simulink model "vardownsampler"  (Simulink 7.3)
settings: Solver=VariableStepDiscrete  StartTime=0.0  StopTime=simTime*SampleTime  RelTol=1e-3
PreLoadFcn:
  | setup_vardownsampler
InitFcn:
  | setup_vardownsampler
values from neighbouring files (symbols this model uses):
  accumOutShift = [1 4 3 2 4]    [setup_vardownsampler.m]    (also in setup_vardownsamplerL8.m = [3 3 2 2 2])
  accumOutWidth = dataWidth + ceil(log2(Rmax))+0    [setup_vardownsampler.m]    (also in setup_vardownsamplerL8.m)
  adderOutShift = 4*ones(1,numRates)    [setup_vardownsampler.m]    (also in setup_vardownsamplerL8.m = 3*ones(1,numRates))
  adderOutWidth = dataWidth + coeffWidth + ceil(log2(L))    [setup_vardownsampler.m]    (also in setup_vardownsamplerL8.m)
  addrWidth = max(1,ceil(log2(Rmax)))    [setup_vardownsampler.m]    (also in setup_vardownsamplerL8.m)
  ChanCount = 16    [setup_vardownsampler.m]    (also in setup_vardownsamplerL8.m = 1)
  ChanCycleCount = ceil(ChanCount/ChanWireCount)    [setup_vardownsampler.m]    (also in setup_vardownsamplerL8.m)
  ChanWireCount = ceil(ChanCount/Period)    [setup_vardownsampler.m]    (also in setup_vardownsamplerL8.m)
  coeffWidth = 16    [setup_vardownsampler.m]    (also in setup_vardownsamplerL8.m)
  dataWidth = 16    [setup_vardownsampler.m]    (also in setup_vardownsamplerL8.m)
  FirAddr = AccumOutScale + 1    (= 4)    [setup_vardownsampler.m]    (also in setup_vardownsamplerL8.m)
  hmatrix = zeros(2*Rmax, L)    [setup_vardownsampler.m]    (also in setup_vardownsamplerL8.m)
  memAddrWidth = max(1,ceil(log2(Nmax)))    [setup_vardownsampler.m]    (also in setup_vardownsamplerL8.m)
  Nmax = Period*Rmax    [setup_vardownsampler.m]    (also in setup_vardownsamplerL8.m)
  Period = floor(ClockRate / SampleRate)    [setup_vardownsampler.m]    (also in setup_vardownsamplerL8.m)
  R = [1 2 5 8 2]    [setup_vardownsampler.m]    (also in setup_vardownsamplerL8.m = [4 5 7 8 9])
  RateWidth = ceil(log2(Rmax))+1    [setup_vardownsampler.m]    (also in setup_vardownsamplerL8.m)
  resetCntWidth = max(1,ceil(log2(Nmax)))    [setup_vardownsampler.m]    (also in setup_vardownsamplerL8.m)
  Rmax = 16    [setup_vardownsampler.m]    (also in setup_vardownsamplerL8.m = 20)
  SampleTime = 1    [setup_vardownsampler.m]    (also in setup_vardownsamplerL8.m)
undefined symbols (not defined in the file or in its folder): AdvDSPBChannelOutDisplay, AdvDSPBDMemDisplay, bank1, bank2, c4, c5, c6, c7, c8, c9, dpoly, dspba_ChannelInVis, dspba_ChannelOutVis, dspba_internal_get_channel_ports, evalAionMaskParam, hmatrix0, hmatrix1, hmatrix2, hmatrix3, latency, primtype, UseDontCare, value
libraries: DSPBAPrim x314, DSPBAModelBus x24, simulink x12, DSPBABase x6
(part 1 of 4)
Description:
  | This model shows how to use the primitive blocks to build a variable integer rate decimation FIR filter. The model has the following features:
  | •Support arbitrary integer decimation rate (including the cases without rate change), arbitrary number of channels and arbitrary clock rate and input sample rate, as long as the clock rate is high enough to process all channels in a single data path (i.e. no hardware duplication).
  | •Support run time reconfiguration of decimation rate.
  | •Use of two memory banks for filter coefficients storage instead of pre-storing coefficients for all rates in memory.  Update one memory bank while the design is reading coefficients from the other bank.
  | •Real time control of scaling in the FIR data path.
  | 
  | The model will generate RTL that can be used in the third party tools.
  | 
  | The parameters for the system can be modified in the file setup_vardownsampleri.m which can be accessed from the Edit Params icon.
settings Model: Creator=sichou  LastModifiedBy=xdong
settings OptimizationCC: InitFltsAndDblsToZero=on
settings DebuggingCC: SaveWithParameterizedLinksMsg=none  SignalResolutionControl=TryResolveAllWithWarning  MultiTaskDSMMsg=warning  MultiTaskCondExecSysMsg=none  StrictBusMsg=None  LoggingUnavailableSignals=none
settings RTWCC: IncludeERTFirstTime=on
settings GRTTargetCC: TargetFcnLib=ansi_tfl_tmw.mat

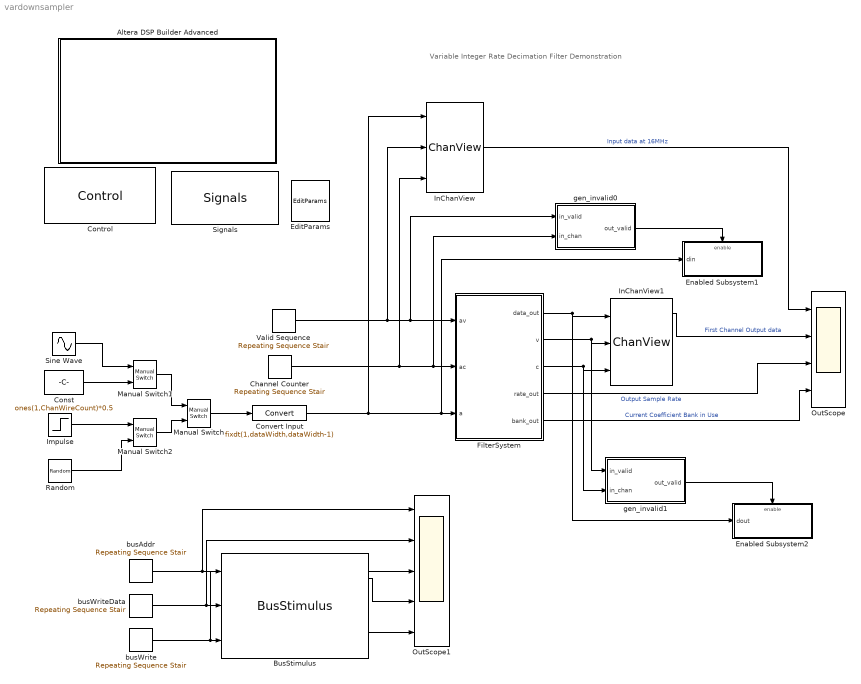
== system vardownsampler ==
  note: Variable Integer Rate Decimation Filter Demonstration
  Altera DSP Builder Advanced : Subsystem
      settings: OpenFcn=web('http://www.altera.com', '-new');
      mask Type: DSP Builder Advanced Blockset Ignored Block
      mask Display: image(imread('alteralogo.tif'));
  BusStimulus : DSPBAModelBus/BusStimulus  SampleTime=-1  version=20090407
  Channel Counter : simulink/Sources/Repeating Sequence Stair  SystemSampleTime=-1  OutValues=[0:ChanCycleCount-1 zeros(1,Period-ChanCycleCount)]  tsamp=SampleTime  OutMin=[]  OutMax=[]  OutDataTypeStr=uint(8)  OutputDataTypeScalingMode=Specify via dialog  OutDataType=uint(8)  ConRadixGroup=Best Precision: Vector-wise  OutScaling=2^-12
  Const : Constant  Value=ones(1,ChanWireCount)*0.5  OutDataType=sfix(16)  OutScaling=2^0
  Control : DSPBABase/Control  generate=off  destination=../rtl  language=VHDL  autotestbench=off  signaldepth=2  coveragetestbench=off  logs=off  spacewidth=2  spacenum=2  addrwidth=16  datawidth=32  dataendian=Big Endian  hierarchicalnames=on  ramThresholdBits=-1  distRamThresholdBits=-1  mlabThresholdBits=-1  hardMultiplierThresholdLuts=-1  version=20090407
  Convert Input : DataTypeConversion  OutDataTypeMode=Specify via dialog  OutDataType=fixdt(1,dataWidth,dataWidth-1)  OutDataTypeStr=fixdt(1,dataWidth,dataWidth-1)  SaturateOnIntegerOverflow=on
  EditParams : DSPBABase/EditParams  SystemSampleTime=-1  version=20090407
  Enabled Subsystem1 : Subsystem  TreatAsAtomicUnit=on
  Enabled Subsystem2 : Subsystem  TreatAsAtomicUnit=on
  FilterSystem : Subsystem
  Impulse : Step  Time=ones(1, ChanWireCount)  Before=1  After=0  SampleTime=SampleTime
  InChanView : DSPBABase/ChanView  nchans=ChanCount  chan_vector=0  latency=0  version=20090407
  InChanView1 : DSPBABase/ChanView  nchans=ChanCount  chan_vector=0:ChanCount-1  latency=0  version=20090407
  Manual Switch : simulink/Signal Routing/Manual Switch  SystemSampleTime=-1  sw=1  action=0  varsize=off
  Manual Switch1 : simulink/Signal Routing/Manual Switch  SystemSampleTime=-1  sw=1  action=0  varsize=off
  Manual Switch2 : simulink/Signal Routing/Manual Switch  SystemSampleTime=-1  sw=0  action=0  varsize=off
  OutScope : Scope  NumInputPorts=4
      settings: TimeRange=20000  YMin=-1~-0.5~-5~-5  YMax=1~0.5~5~5  SaveName=iout  DataFormat=Structure
  OutScope1 : Scope  NumInputPorts=5
      settings: TimeRange=20000  YMin=-1~-0.5~-5~-5~-5  YMax=1~0.5~5~5~5  SaveName=iout1  DataFormat=Structure
  Random : RandomNumber  Seed=1:ChanWireCount  SampleTime=SampleTime
  Signals : DSPBABase/Signals  SystemSampleTime=-1  clk=clk  freq=ClockRate  margin=ClockMargin  rst=areset  rstactive=High  bus=bus  enbusclock=on  busfreq=BusClockRate  bussync=on  version=20090407
  Sine Wave : Sin  SineType=Sample based  Amplitude=ones(1,ChanWireCount)*(2^17-2)/(2^17)  Bias=0  Frequency=(2 * pi) / ( 4 * 2^24 / floor(2^24 * 0.051))  Phase=0  Samples=Rmax*50  SampleTime=SampleTime  Offset=0
  Valid Sequence : simulink/Sources/Repeating Sequence Stair  SystemSampleTime=-1  OutValues=v_in  tsamp=SampleTime  OutMin=[]  OutMax=[]  OutDataTypeStr=Inherit: Inherit via back propagation  OutDataType=float('double')  ConRadixGroup=Best Precision: Vector-wise  OutScaling=2^-12
  busAddr : simulink/Sources/Repeating Sequence Stair  SystemSampleTime=-1  OutValues=busAddr  tsamp=SampleTime  OutMin=[]  OutMax=[]  OutDataTypeStr=uint16  OutputDataTypeScalingMode=uint16  OutDataType=float('double')  ConRadixGroup=Best Precision: Vector-wise  OutScaling=2^-12
  busWrite : simulink/Sources/Repeating Sequence Stair  SystemSampleTime=-1  OutValues=busWrite  tsamp=SampleTime  OutMin=[]  OutMax=[]  OutDataTypeStr=Inherit: Inherit via back propagation  OutDataType=ufix(1)  ConRadixGroup=Best Precision: Vector-wise  OutScaling=[]
  busWriteData : simulink/Sources/Repeating Sequence Stair  SystemSampleTime=-1  OutValues=busWriteData  tsamp=SampleTime  OutMin=[]  OutMax=[]  OutDataTypeStr=uint32  OutputDataTypeScalingMode=uint32  OutDataType=fixdt(1,32,2^0,0)  ConRadixGroup=Best Precision: Vector-wise  OutScaling=[]
  gen_invalid0 : Subsystem
  gen_invalid1 : Subsystem
  wires:
  Manual Switch2/1 -> Manual Switch/2
  Impulse/1 -> Manual Switch2/1
  Random/1 -> Manual Switch2/2
  Manual Switch/1 -> Convert Input/1
  Manual Switch1/1 -> Manual Switch/1
  Sine Wave/1 -> Manual Switch1/1
  Const/1 -> Manual Switch1/2
  Convert Input/1 -> InChanView/1, Enabled Subsystem1/1(din), FilterSystem/3(a)
  Channel Counter/1 -> InChanView/3, FilterSystem/2(ac), gen_invalid0/2(in_chan)
  Valid Sequence/1 -> InChanView/2, FilterSystem/1(av), gen_invalid0/1(in_valid)
  gen_invalid1/1(out_valid) -> Enabled Subsystem2/Enable
  gen_invalid0/1(out_valid) -> Enabled Subsystem1/Enable
  busAddr/1 -> BusStimulus/1, OutScope1/1
  busWriteData/1 -> BusStimulus/2, OutScope1/2
  busWrite/1 -> BusStimulus/3, OutScope1/3
  InChanView/1 -> OutScope/1  "Input data at 16MHz"
  InChanView1/1 -> OutScope/2  "First Channel Output data"
  BusStimulus/1 -> OutScope1/4
  BusStimulus/2 -> OutScope1/5
  FilterSystem/1(data_out) -> InChanView1/1, Enabled Subsystem2/1(dout)
  FilterSystem/2(v) -> InChanView1/2, gen_invalid1/1(in_valid)
  FilterSystem/3(c) -> InChanView1/3, gen_invalid1/2(in_chan)
  FilterSystem/4(rate_out) -> OutScope/3  "Output Sample Rate"
  FilterSystem/5(bank_out) -> OutScope/4  "Current Coefficient Bank in Use"

== system vardownsampler/Altera DSP Builder Advanced ==

== system vardownsampler/Enabled Subsystem1 ==
  din : Inport  OutDataType=fixdt(1, 16)  OutScaling=2^0
  Enable : EnablePort
  To Workspace : ToWorkspace  VariableName=din  SampleTime=SampleTime  SaveFormat=Array
  wires:
  din/1 -> To Workspace/1

== system vardownsampler/Enabled Subsystem2 ==
  dout : Inport  OutDataType=fixdt(1, 16)  OutScaling=2^0
  Enable : EnablePort
  To Workspace : ToWorkspace  VariableName=dout  SampleTime=SampleTime  SaveFormat=Array
  wires:
  dout/1 -> To Workspace/1

== system vardownsampler/FilterSystem ==
  av : Inport  OutDataType=sfix(16)  OutScaling=2^0
  ac : Inport  Port=2  OutDataType=sfix(16)  OutScaling=2^0
  a : Inport  Port=3  OutDataType=sfix(16)  OutScaling=2^0
  Device : DSPBABase/Device  SystemSampleTime=-1  family=Stratix IV  deviceMember=Stratix IV E  stratix4device=Stratix IV E  hardcopy4device=HardCopy IV E  device=AUTO  speed=-2  stratixSpeed=-5  stratix2Speed=-3  stratix3Speed=-2  stratix4gxSpeed=-2  stratix4gtSpeed=-1  cyclone2Speed=-6  cyclone3Speed=-6  arria2Speed=-4  ecp2Speed=-7  version=20090914
  FIRSubsystem : Subsystem
  Rate : DSPBAModelBus/RegField  reg_name=RateAddr  reg_rwmode=Read/Write  reg_msb=RateWidth-1  reg_lsb=0  reg_type=ufix(RateWidth)  reg_scale=1  reg_init=R(1)  reg_desc=Decimation Rate  reg_modal=off  reg_desc0=0  reg_desc1=0  reg_desc2=0  reg_desc3=0  reg_desc4=0  reg_desc5=0  reg_desc6=0  reg_desc7=0  reg_addr=1  SampleTime=SampleTime  version=20090407
  Terminator : Terminator
  coefficients_gen : Subsystem
  gen_addr_control : Subsystem
  data_out : Outport  OutDataType=sfix(16)  OutScaling=2^0
  v : Outport  Port=2  OutDataType=sfix(16)  OutScaling=2^0
  c : Outport  Port=3  OutDataType=sfix(16)  OutScaling=2^0
  rate_out : Outport  Port=4  OutDataType=sfix(16)  OutScaling=2^0
  bank_out : Outport  Port=5  OutDataType=sfix(16)  OutScaling=2^0
  wires:
  Rate/1 -> gen_addr_control/3(rate_in)
  av/1 -> gen_addr_control/1(v)
  ac/1 -> gen_addr_control/2(c)
  a/1 -> gen_addr_control/4(data_in)
  gen_addr_control/1(qv) -> coefficients_gen/1(v)
  gen_addr_control/2(qc) -> coefficients_gen/2(c)
  gen_addr_control/3(coeff_addr) -> coefficients_gen/3(coeff_addr)
  coefficients_gen/3(coeff) -> FIRSubsystem/3(coeff)
  coefficients_gen/1(qv) -> FIRSubsystem/1(dv)
  coefficients_gen/2(qc) -> FIRSubsystem/2(dc)
  gen_addr_control/5(mem_addr) -> coefficients_gen/5(mem_addr)
  gen_addr_control/6(data_out) -> coefficients_gen/6(data_in)
  gen_addr_control/7(rate_out) -> coefficients_gen/7(rate_in)
  gen_addr_control/8(outvalid) -> coefficients_gen/8(outvalid_in)
  coefficients_gen/4(mem_addr_out) -> FIRSubsystem/4(mem_addr)
  coefficients_gen/5(data_out) -> FIRSubsystem/5(data_in)
  coefficients_gen/6(rate_out) -> FIRSubsystem/6(rate_in)
  coefficients_gen/7(outvalid) -> FIRSubsystem/7(outvalid_in)
  FIRSubsystem/4(rate_out) -> rate_out/1
  FIRSubsystem/3(data_out) -> data_out/1
  FIRSubsystem/2(c) -> c/1
  FIRSubsystem/5(valid_out) -> v/1
  FIRSubsystem/1(v) -> Terminator/1
  gen_addr_control/4(coffset) -> coefficients_gen/4(coffset)
  coefficients_gen/8(bank) -> FIRSubsystem/8(bank_in)
  FIRSubsystem/6(bank_out) -> bank_out/1

== system vardownsampler/gen_invalid0 ==
  note: Generate valid signal for the 1st channel
  in_valid : Inport
  in_chan : Inport  Port=2
  Bitwise Operator : simulink/Logic and Bit Operations/Bitwise Operator  logicop=AND  UseBitMask=off  NumInputPorts=2  BitMask=bin2dec('11011001')  BitMaskRealWorld=Stored Integer
  Compare To Constant : simulink/Logic and Bit Operations/Compare To Constant  SystemSampleTime=-1  relop===  const=0  LogicOutDataTypeMode=boolean  ZeroCross=off
  out_valid : Outport
  wires:
  Compare To Constant/1 -> Bitwise Operator/2
  in_valid/1 -> Bitwise Operator/1
  in_chan/1 -> Compare To Constant/1
  Bitwise Operator/1 -> out_valid/1

== system vardownsampler/gen_invalid1 ==
  note: Generate valid signal for the 1st channel
  in_valid : Inport
  in_chan : Inport  Port=2
  Bitwise Operator : simulink/Logic and Bit Operations/Bitwise Operator  logicop=AND  UseBitMask=off  NumInputPorts=2  BitMask=bin2dec('11011001')  BitMaskRealWorld=Stored Integer
  Compare To Constant : simulink/Logic and Bit Operations/Compare To Constant  SystemSampleTime=-1  relop===  const=0  LogicOutDataTypeMode=boolean  ZeroCross=off
  out_valid : Outport
  wires:
  in_chan/1 -> Compare To Constant/1
  Compare To Constant/1 -> Bitwise Operator/2
  in_valid/1 -> Bitwise Operator/1
  Bitwise Operator/1 -> out_valid/1

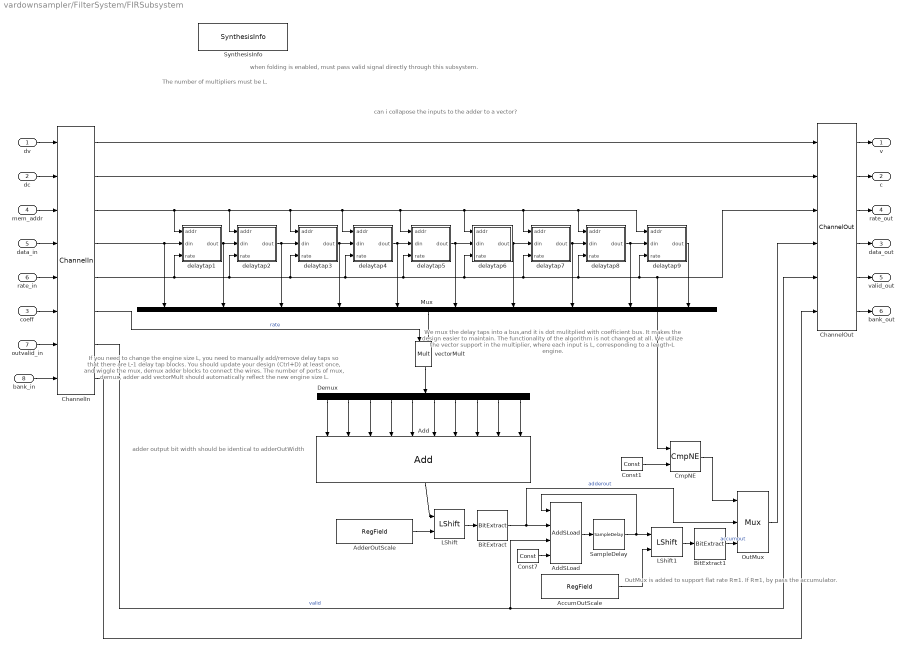
== system vardownsampler/FilterSystem/FIRSubsystem ==
  note: adder output bit width should be identical to adderOutWidth
  note: when folding is enabled, must pass valid signal directly through this subsystem.
  note: The number of multipliers must be L.
  note: can i collapose the inputs to the adder to a vector?
  note: We mux the delay taps into a bus,and it is dot mulitplied
      | with coefficient bus.  It makes the design easier to maintain.
      | The functionality of the algorithm is not changed at all.
      | We utilize the vector support in the multiplier, where
      | each input is L, corresponding to a length-L engine.
  note: If you need to change the engine size L,
      | you need to manually add/remove delay taps
      | so that there are L-1 delay tap blocks.  You should
      | update your design (Ctrl+D) at least once, and
      | wiggle the mux, demux adder blocks to connect
      |  the wires.  The number of ports of mux, demux, adder
      | add vectorMult should automatically reflect the new
      | engine size L.
  note: OutMux is added to support flat rate R=1.
      | If R=1, by pass the accumulator.
  dv : Inport  OutDataType=sfix(16)  OutScaling=2^0
  dc : Inport  Port=2  OutDataType=sfix(16)  OutScaling=2^0
  coeff : Inport  Port=3  OutDataType=sfix(16)  OutScaling=2^0
  mem_addr : Inport  Port=4  OutDataType=sfix(16)  OutScaling=2^0
  data_in : Inport  Port=5  OutDataType=sfix(16)  OutScaling=2^0
  rate_in : Inport  Port=6  OutDataType=sfix(16)  OutScaling=2^0
  outvalid_in : Inport  Port=7  OutDataType=sfix(16)  OutScaling=2^0
  bank_in : Inport  Port=8  OutDataType=sfix(16)  OutScaling=2^0
  AccumOutScale : DSPBAModelBus/RegField  reg_name=AccumOutScale  reg_rwmode=Read/Write  reg_msb=15  reg_lsb=0  reg_type=ufix(16)  reg_scale=1  reg_init=accumOutShift(1)  reg_desc=Left shift value forthe final accumulator output  reg_modal=off  reg_desc0=0  reg_desc1=0  reg_desc2=0  reg_desc3=0  reg_desc4=0  reg_desc5=0  reg_desc6=0  reg_desc7=0  reg_addr=3  SampleTime=-1  version=20090407
  Add : DSPBAPrim/Add  primtype=add  nInputs=evalAionMaskParam(gcb,'value',1)  nOutputs=1  omode=Inherit via internal rule with word growth  otype=sfix(adderOutWidth)  scale=2^-(adderOutWidth-1)  rndmethod=Unbiased  factor=1  satmethod=Symmetric  shift_vec=[0 1 2 -1]  value=L  inPortNames=[' '; ' ';]  outPortNames=[' ']  image=dspba_prim.jpg  text=fprintf('+');  style=Optimised  visibilities=1032  version=20090731
  AddSLoad : DSPBAPrim/AddSLoad  primtype=addsload  nInputs=4  nOutputs=1  omode=Specify via dialog  otype=sfix(accumOutWidth)  scale=2^-(dataWidth-1)  rndmethod=Unbiased  factor=1  satmethod=Symmetric  shift_vec=[0 1 2 -1]  value=0  inPortNames=['+'; '+'; 's'; 'v']  outPortNames=[' ']  image=dspba_prim.jpg  text=fprintf('+');  style=Optimised  visibilities=8  version=20090407
  AdderOutScale : DSPBAModelBus/RegField  reg_name=AdderOutScale  reg_rwmode=Read/Write  reg_msb=15  reg_lsb=0  reg_type=ufix(16)  reg_scale=1  reg_init=adderOutShift(1)  reg_desc=Left shift value forthe final adder output  reg_modal=off  reg_desc0=0  reg_desc1=0  reg_desc2=0  reg_desc3=0  reg_desc4=0  reg_desc5=0  reg_desc6=0  reg_desc7=0  reg_addr=2  SampleTime=-1  version=20090407
  BitExtract : DSPBAPrim/BitExtract  primtype=bitextract  nInputs=1  nOutputs=1  omode=Specify via dialog  otype=sfix(dataWidth)  scale=2^-(dataWidth-1)  rndmethod=Unbiased  factor=1  satmethod=Symmetric  shift_vec=[0 1 2 -1]  value=adderOutWidth - dataWidth  inPortNames=[' '; ' ';]  outPortNames=[' ']  image=dspba_prim.jpg  text=fprintf('..%d', value);  style=Optimised  visibilities=8 + 1024  version=20090407
  BitExtract1 : DSPBAPrim/BitExtract  primtype=bitextract  nInputs=1  nOutputs=1  omode=Specify via dialog  otype=sfix(dataWidth)  scale=2^-(dataWidth-1)  rndmethod=Unbiased  factor=1  satmethod=Symmetric  shift_vec=[0 1 2 -1]  value=accumOutWidth - dataWidth  inPortNames=[' '; ' ';]  outPortNames=[' ']  image=dspba_prim.jpg  text=fprintf('..%d', value);  style=Optimised  visibilities=8 + 1024  version=20090407
  ChannelIn : DSPBAPrim/ChannelIn  primtype=channelin  nInputs=dspba_internal_get_channel_ports(gcb)  nOutputs=dspba_internal_get_channel_ports(gcb)  omode=Inherit via internal rule  otype=sfix(16)  scale=2^-15  rndmethod=Unbiased  factor=1  satmethod=Symmetric  shift_vec=[0 1 2 -1]  value=6  inPortNames=['v'; 'c'; '0'; '1'; '2'; '3'; '4'; '5'; '6'; '7'; '8'; '9'; 'A'; 'B'; 'D'; 'E'; 'F'; 'G'; 'H'; 'I'; 'J'; 'K'; 'L'; 'M'; 'N'; 'O'; 'P'; 'Q'; 'R'; 'S'; 'T'; 'U'; 'W'; 'X'; 'Y'; 'Z']  outPortNames=['v'; 'c'; '0'; '1'; '2'; '3'; '4'; '5'; '6'; '7'; '8'; '9'; 'A'; 'B'; 'D'; 'E'; 'F'; 'G'; 'H'; 'I'; 'J'; 'K'; 'L'; 'M'; 'N'; 'O'; 'P'; 'Q'; 'R'; 'S'; 'T'; 'U'; 'W'; 'X'; 'Y'; 'Z']  image=dspba_prim.jpg  text=fprintf('In');  style=Optimised  dataSignals=6  foldingEnabled=off  channels=ChanCount  sampleRate=SampleRate  visibilities=dspba_ChannelInVis(gcb)  version=20090408
  ChannelOut : DSPBAPrim/ChannelOut  primtype=channelout  nInputs=dspba_internal_get_channel_ports(gcb)  nOutputs=dspba_internal_get_channel_ports(gcb)  omode=Inherit via internal rule  otype=sfix(16)  scale=2^-15  rndmethod=Unbiased  factor=1  satmethod=Symmetric  shift_vec=[0 1 2 -1]  value=4  inPortNames=['v'; 'c'; '0'; '1'; '2'; '3'; '4'; '5'; '6'; '7'; '8'; '9'; 'A'; 'B'; 'D'; 'E'; 'F'; 'G'; 'H'; 'I'; 'J'; 'K'; 'L'; 'M'; 'N'; 'O'; 'P'; 'Q'; 'R'; 'S'; 'T'; 'U'; 'W'; 'X'; 'Y'; 'Z']  outPortNames=['v'; 'c'; '0'; '1'; '2'; '3'; '4'; '5'; '6'; '7'; '8'; '9'; 'A'; 'B'; 'D'; 'E'; 'F'; 'G'; 'H'; 'I'; 'J'; 'K'; 'L'; 'M'; 'N'; 'O'; 'P'; 'Q'; 'R'; 'S'; 'T'; 'U'; 'W'; 'X'; 'Y'; 'Z']  image=dspba_prim.jpg  text=fprintf('Out%s', AdvDSPBChannelOutDisplay(latency));  style=Optimised  dataSignals=4  foldingEnabled=off  channels=ChanCount  sampleRate=SampleRate  visibilities=dspba_ChannelOutVis(gcb)  latency=0  version=20090408
  CmpNE : DSPBAPrim/CmpNE  primtype=cmpne  nInputs=2  nOutputs=1  omode=boolean  otype=sfix(16)  scale=2^-15  rndmethod=Unbiased  factor=1  satmethod=Symmetric  shift_vec=[0 1 2 -1]  value=0  inPortNames=[' '; ' ';]  outPortNames=[' ']  image=dspba_prim.jpg  text=fprintf('~=');  style=Optimised  visibilities=0  version=20090407
  Const1 : DSPBAPrim/Const  primtype=const  nInputs=0  nOutputs=1  omode=Specify via dialog  otype=ufix(RateWidth)  scale=1  rndmethod=Unbiased  factor=1  satmethod=Symmetric  shift_vec=[0 1 2 -1]  value=1  inPortNames=['+'; '+';]  outPortNames=[' ']  image=dspba_prim.jpg  text=fprintf('%s', num2str(value));  style=Optimised  visibilities=8 + 1024  version=20090407
  Const7 : DSPBAPrim/Const  primtype=const  nInputs=0  nOutputs=1  omode=Specify via dialog  otype=uint(accumOutWidth)  scale=1  rndmethod=Unbiased  factor=1  satmethod=Symmetric  shift_vec=[0 1 2 -1]  value=0  inPortNames=['+'; '+';]  outPortNames=[' ']  image=dspba_prim.jpg  text=fprintf('%s', num2str(value));  style=Optimised  visibilities=8 + 1024  version=20090407
  Demux : Demux  Outputs=L
  LShift : DSPBAPrim/LShift  primtype=lshift  nInputs=2  nOutputs=1  omode=Specify via dialog  otype=sfix(adderOutWidth)  scale=1  rndmethod=Unbiased  factor=1  satmethod=Symmetric  shift_vec=[0 1 2 -1]  value=0  inPortNames=['a'; 'b';]  outPortNames=[' ']  image=dspba_prim.jpg  text=fprintf('a << b');  style=Optimised  visibilities=8  version=20090407
  LShift1 : DSPBAPrim/LShift  primtype=lshift  nInputs=2  nOutputs=1  omode=Specify via dialog  otype=sfix(accumOutWidth)  scale=1  rndmethod=Unbiased  factor=1  satmethod=Symmetric  shift_vec=[0 1 2 -1]  value=0  inPortNames=['a'; 'b';]  outPortNames=[' ']  image=dspba_prim.jpg  text=fprintf('a << b');  style=Optimised  visibilities=8  version=20090407
  Mux : Mux  Inputs=L
  OutMux : DSPBAPrim/Mux  primtype=mux  nInputs=evalAionMaskParam(gcb,'value',1)+1  nOutputs=1  omode=Inherit via internal rule  otype=sfix(16)  scale=2^-15  rndmethod=Unbiased  factor=1  satmethod=Symmetric  shift_vec=[0 1 2 -1]  value=2  inPortNames=['s'; 'd0'; 'd1'; 'd2'; 'd3'; 'd4'; 'd5'; 'd6'; 'd7'; 'd8'; 'd9';]  outPortNames=[' ']  image=dspba_prim.jpg  text=fprintf('%s', primtype);  style=Optimised  visibilities=1032  version=20090623
  SampleDelay : DSPBAPrim/SampleDelay  primtype=sampdelay  nInputs=1  nOutputs=1  omode=Inherit via internal rule  otype=sfix(accumOutWidth)  scale=2^-(dataWidth - 1)  rndmethod=Unbiased  factor=1  satmethod=Symmetric  shift_vec=[0 1 2 -1]  value=Period  inPortNames=[' '; ' ';]  outPortNames=[' ']  image=dspba_prim.jpg  text=dpoly(1, eye(1,value+1), 'z')  style=Optimised  visibilities=8 + 1024  version=20090407
  SynthesisInfo : DSPBAPrim/SynthesisInfo  primtype=synthinfo  nInputs=0  nOutputs=0  omode=Inherit via internal rule  otype=sfix(16)  scale=2^-15  rndmethod=Truncate  factor=1  satmethod=Symmetric  shift_vec=[0 1 2 -1]  value=99  inPortNames=[' '; ' ';]  outPortNames=[' ']  image=dspba_prim_ctrl.jpg  text=fprintf('Style=%s', style);  style=Scheduled  visibilities=32768  constraintInUse=off  constraintRelation=>  constraintLimit=2  version=20090407
  delaytap1 : Subsystem
  delaytap2 : Subsystem
  delaytap3 : Subsystem
  delaytap4 : Subsystem
  delaytap5 : Subsystem
  delaytap6 : Subsystem
  delaytap7 : Subsystem
  delaytap8 : Subsystem
  delaytap9 : Subsystem
  vectorMult : DSPBAPrim/Mult  primtype=mult  nInputs=2  nOutputs=1  omode=Inherit via internal rule  otype=sfix(16)  scale=2^-15  rndmethod=Unbiased  factor=1  satmethod=Symmetric  shift_vec=[0 1 2 -1]  value=0  inPortNames=[' '; ' ';]  outPortNames=[' ']  image=dspba_prim.jpg  text=fprintf('X');  style=Optimised  visibilities=8  version=20090407
  v : Outport  OutDataType=sfix(16)  OutScaling=2^0
  c : Outport  Port=2  OutDataType=sfix(16)  OutScaling=2^0
  data_out : Outport  Port=3  OutDataType=sfix(16)  OutScaling=2^0
  rate_out : Outport  Port=4  OutDataType=sfix(16)  OutScaling=2^0
  valid_out : Outport  Port=5  OutDataType=sfix(16)  OutScaling=2^0
  bank_out : Outport  Port=6  OutDataType=sfix(16)  OutScaling=2^0
  wires:
  dv/1 -> ChannelIn/1
  dc/1 -> ChannelIn/2
  ChannelIn/2 -> ChannelOut/2
  ChannelOut/1 -> v/1
  ChannelOut/2 -> c/1
  LShift/1 -> BitExtract/1
  data_in/1 -> ChannelIn/4
  mem_addr/1 -> ChannelIn/3
  ChannelIn/3 -> delaytap8/1(addr), delaytap9/1(addr), delaytap7/1(addr), delaytap6/1(addr), delaytap5/1(addr), delaytap4/1(addr), delaytap3/1(addr), delaytap2/1(addr), delaytap1/1(addr)
  ChannelIn/4 -> Mux/1, delaytap1/2(din)
  Add/1 -> LShift/1
  AdderOutScale/1 -> LShift/2
  ChannelIn/1 -> ChannelOut/1
  ChannelIn/7 -> ChannelOut/5, AddSLoad/3  "valid"
  ChannelOut/5 -> valid_out/1
  delaytap1/1(dout) -> Mux/2, delaytap2/2(din)
  delaytap2/1(dout) -> delaytap3/2(din), Mux/3
  delaytap3/1(dout) -> Mux/4, delaytap4/2(din)
  delaytap4/1(dout) -> delaytap5/2(din), Mux/5
  delaytap5/1(dout) -> delaytap6/2(din), Mux/6
  delaytap6/1(dout) -> delaytap7/2(din), Mux/7
  delaytap7/1(dout) -> delaytap8/2(din), Mux/8
  delaytap8/1(dout) -> delaytap9/2(din), Mux/9
  BitExtract/1 -> AddSLoad/2, OutMux/2  "adderout"
  AddSLoad/1 -> SampleDelay/1
  SampleDelay/1 -> AddSLoad/1, LShift1/1
  Const7/1 -> AddSLoad/4
  LShift1/1 -> BitExtract1/1
  AccumOutScale/1 -> LShift1/2
  delaytap9/1(dout) -> Mux/10
  Mux/1 -> vectorMult/2
  coeff/1 -> ChannelIn/6
  rate_in/1 -> ChannelIn/5
  ChannelIn/5 -> delaytap3/3(rate), ChannelOut/3, CmpNE/1, delaytap9/3(rate), delaytap8/3(rate), delaytap7/3(rate), delaytap6/3(rate), delaytap5/3(rate), delaytap4/3(rate), delaytap2/3(rate), delaytap1/3(rate)
  ChannelIn/6 -> vectorMult/1  "rate"
  outvalid_in/1 -> ChannelIn/7
  vectorMult/1 -> Demux/1
  Demux/1 -> Add/1
  Demux/2 -> Add/2
  Demux/3 -> Add/3
  Demux/4 -> Add/4
  Demux/5 -> Add/5
  Demux/6 -> Add/6
  Demux/7 -> Add/7
  Demux/8 -> Add/8
  Demux/9 -> Add/9
  Demux/10 -> Add/10
  ChannelOut/3 -> rate_out/1
  ChannelOut/4 -> data_out/1
  BitExtract1/1 -> OutMux/3  "accumout"
  Const1/1 -> CmpNE/2
  CmpNE/1 -> OutMux/1
  OutMux/1 -> ChannelOut/4
  bank_in/1 -> ChannelIn/8
  ChannelIn/8 -> ChannelOut/6
  ChannelOut/6 -> bank_out/1

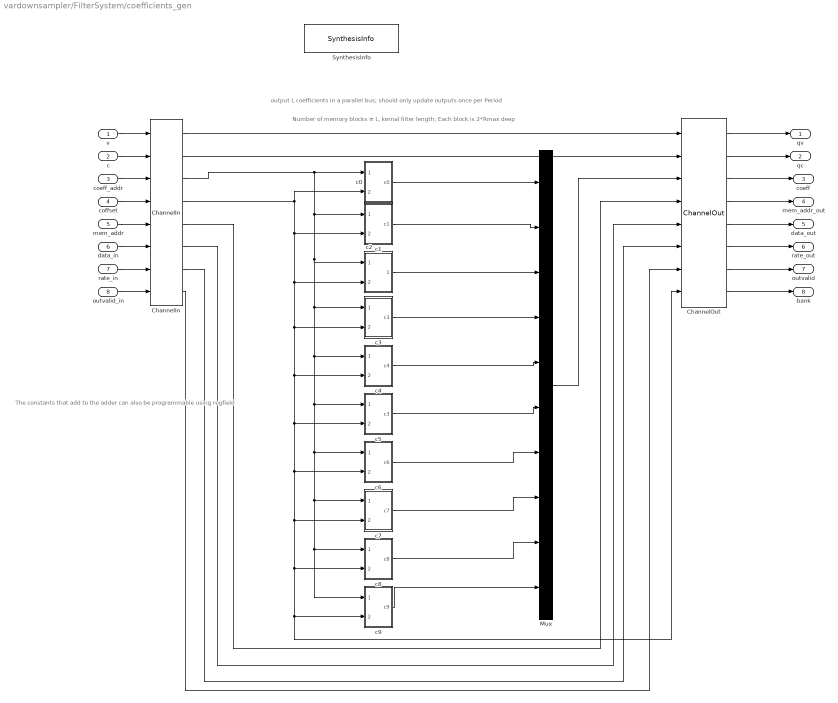
== system vardownsampler/FilterSystem/coefficients_gen ==
  note: output L coefficients in a parallel bus; should only update outputs once per Period
  note: The constants that add to the adder can also
      | be programmable using regfield
  note: Number of memory blocks = L, kernal filter length;
      | Each block is 2*Rmax deep
  v : Inport  OutDataType=sfix(16)  OutScaling=2^0
  c : Inport  Port=2  OutDataType=sfix(16)  OutScaling=2^0
  coeff_addr : Inport  Port=3  OutDataType=sfix(16)  OutScaling=2^0
  coffset : Inport  Port=4  OutDataType=sfix(16)  OutScaling=2^0
  mem_addr : Inport  Port=5  OutDataType=sfix(16)  OutScaling=2^0
  data_in : Inport  Port=6  OutDataType=sfix(16)  OutScaling=2^0
  rate_in : Inport  Port=7  OutDataType=sfix(16)  OutScaling=2^0
  outvalid_in : Inport  Port=8  OutDataType=sfix(16)  OutScaling=2^0
  ChannelIn : DSPBAPrim/ChannelIn  primtype=channelin  nInputs=dspba_internal_get_channel_ports(gcb)  nOutputs=dspba_internal_get_channel_ports(gcb)  omode=Inherit via internal rule  otype=sfix(16)  scale=2^-15  rndmethod=Unbiased  factor=1  satmethod=Symmetric  shift_vec=[0 1 2 -1]  value=6  inPortNames=['v'; 'c'; '0'; '1'; '2'; '3'; '4'; '5'; '6'; '7'; '8'; '9'; 'A'; 'B'; 'D'; 'E'; 'F'; 'G'; 'H'; 'I'; 'J'; 'K'; 'L'; 'M'; 'N'; 'O'; 'P'; 'Q'; 'R'; 'S'; 'T'; 'U'; 'W'; 'X'; 'Y'; 'Z']  outPortNames=['v'; 'c'; '0'; '1'; '2'; '3'; '4'; '5'; '6'; '7'; '8'; '9'; 'A'; 'B'; 'D'; 'E'; 'F'; 'G'; 'H'; 'I'; 'J'; 'K'; 'L'; 'M'; 'N'; 'O'; 'P'; 'Q'; 'R'; 'S'; 'T'; 'U'; 'W'; 'X'; 'Y'; 'Z']  image=dspba_prim.jpg  text=fprintf('In');  style=Optimised  dataSignals=6  foldingEnabled=off  channels=ChanCount  sampleRate=SampleRate  visibilities=dspba_ChannelInVis(gcb)  version=20090408
  ChannelOut : DSPBAPrim/ChannelOut  primtype=channelout  nInputs=dspba_internal_get_channel_ports(gcb)  nOutputs=dspba_internal_get_channel_ports(gcb)  omode=Inherit via internal rule  otype=sfix(16)  scale=2^-15  rndmethod=Unbiased  factor=1  satmethod=Symmetric  shift_vec=[0 1 2 -1]  value=6  inPortNames=['v'; 'c'; '0'; '1'; '2'; '3'; '4'; '5'; '6'; '7'; '8'; '9'; 'A'; 'B'; 'D'; 'E'; 'F'; 'G'; 'H'; 'I'; 'J'; 'K'; 'L'; 'M'; 'N'; 'O'; 'P'; 'Q'; 'R'; 'S'; 'T'; 'U'; 'W'; 'X'; 'Y'; 'Z']  outPortNames=['v'; 'c'; '0'; '1'; '2'; '3'; '4'; '5'; '6'; '7'; '8'; '9'; 'A'; 'B'; 'D'; 'E'; 'F'; 'G'; 'H'; 'I'; 'J'; 'K'; 'L'; 'M'; 'N'; 'O'; 'P'; 'Q'; 'R'; 'S'; 'T'; 'U'; 'W'; 'X'; 'Y'; 'Z']  image=dspba_prim.jpg  text=fprintf('Out%s', AdvDSPBChannelOutDisplay(latency));  style=Optimised  dataSignals=6  foldingEnabled=off  channels=ChanCount  sampleRate=SampleRate  visibilities=dspba_ChannelOutVis(gcb)  latency=0  version=20090408
  Mux : Mux  Inputs=L
  SynthesisInfo : DSPBAPrim/SynthesisInfo  primtype=synthinfo  nInputs=0  nOutputs=0  omode=Inherit via internal rule  otype=sfix(16)  scale=2^-15  rndmethod=Truncate  factor=1  satmethod=Symmetric  shift_vec=[0 1 2 -1]  value=99  inPortNames=[' '; ' ';]  outPortNames=[' ']  image=dspba_prim_ctrl.jpg  text=fprintf('Style=%s', style);  style=Scheduled  visibilities=32768  constraintInUse=off  constraintRelation=>  constraintLimit=2  version=20090407
  c0 : Subsystem
  c1 : Subsystem
  c2 : Subsystem
  c3 : Subsystem
  c4 : Subsystem
  c5 : Subsystem
  c6 : Subsystem
  c7 : Subsystem
  c8 : Subsystem
  c9 : Subsystem
  qv : Outport  OutDataType=sfix(16)  OutScaling=2^0
  qc : Outport  Port=2  OutDataType=sfix(16)  OutScaling=2^0
  coeff : Outport  Port=3  OutDataType=sfix(16)  OutScaling=2^0
  mem_addr_out : Outport  Port=4  OutDataType=sfix(16)  OutScaling=2^0
  data_out : Outport  Port=5  OutDataType=sfix(16)  OutScaling=2^0
  rate_out : Outport  Port=6  OutDataType=sfix(16)  OutScaling=2^0
  outvalid : Outport  Port=7  OutDataType=sfix(16)  OutScaling=2^0
  bank : Outport  Port=8  OutDataType=sfix(16)  OutScaling=2^0
  wires:
  v/1 -> ChannelIn/1
  c/1 -> ChannelIn/2
  ChannelOut/1 -> qv/1
  ChannelOut/2 -> qc/1
  ChannelIn/1 -> ChannelOut/1
  coeff_addr/1 -> ChannelIn/3
  ChannelIn/2 -> ChannelOut/2
  ChannelOut/3 -> coeff/1
  ChannelIn/3 -> c1/1(addr), c8/1(addr), c9/1(addr), c7/1(addr), c6/1(addr), c5/1(addr), c4/1(addr), c3/1(addr), c2/1(addr), c0/1(addr)
  ChannelOut/4 -> mem_addr_out/1
  ChannelOut/5 -> data_out/1
  ChannelOut/6 -> rate_out/1
  ChannelOut/7 -> outvalid/1
  c0/1(c0) -> Mux/1
  c1/1(c1) -> Mux/2
  c2/1(Out1) -> Mux/3
  c3/1(c3) -> Mux/4
  c4/1(c4) -> Mux/5
  c5/1(c3) -> Mux/6
  c6/1(c6) -> Mux/7
  c7/1(c7) -> Mux/8
  c8/1(c8) -> Mux/9
  c9/1(c9) -> Mux/10
  Mux/1 -> ChannelOut/3
  coffset/1 -> ChannelIn/4
  mem_addr/1 -> ChannelIn/5
  data_in/1 -> ChannelIn/6
  rate_in/1 -> ChannelIn/7
  outvalid_in/1 -> ChannelIn/8
  ChannelIn/4 -> c0/2(offset), c1/2(offset), c2/2(offset), c3/2(offset), c4/2(offset), c5/2(offset), c6/2(offset), c7/2(offset), c8/2(offset), c9/2(offset), ChannelOut/8
  ChannelIn/5 -> ChannelOut/4
  ChannelIn/6 -> ChannelOut/5
  ChannelIn/7 -> ChannelOut/6
  ChannelIn/8 -> ChannelOut/7
  ChannelOut/8 -> bank/1

== system vardownsampler/FilterSystem/gen_addr_control ==
  note: the coefficients address counter should only update contents once per period; it is in the range of [0,R-1]
  note: the memory address counter is updated every cycle; it is in the range of [0, R*Period-1]
  note: When the rate changes, we use a flag signal transig to signal the transition.  transig in turn controls the coefficients address offset.
      | We also force the coefficients counter to reset to zero when the rate changes, so that we start reading coefficients from
      | the start of the other memory bank.
  v : Inport  OutDataType=sfix(16)  OutScaling=2^0
  c : Inport  Port=2  OutDataType=sfix(16)  OutScaling=2^0
  rate_in : Inport  Port=3  OutDataType=sfix(16)  OutScaling=2^0
  data_in : Inport  Port=4  OutDataType=sfix(16)  OutScaling=2^0
  ChannelIn : DSPBAPrim/ChannelIn  primtype=channelin  nInputs=dspba_internal_get_channel_ports(gcb)  nOutputs=dspba_internal_get_channel_ports(gcb)  omode=Inherit via internal rule  otype=sfix(16)  scale=2^-15  rndmethod=Unbiased  factor=1  satmethod=Symmetric  shift_vec=[0 1 2 -1]  value=2  inPortNames=['v'; 'c'; '0'; '1'; '2'; '3'; '4'; '5'; '6'; '7'; '8'; '9'; 'A'; 'B'; 'D'; 'E'; 'F'; 'G'; 'H'; 'I'; 'J'; 'K'; 'L'; 'M'; 'N'; 'O'; 'P'; 'Q'; 'R'; 'S'; 'T'; 'U'; 'W'; 'X'; 'Y'; 'Z']  outPortNames=['v'; 'c'; '0'; '1'; '2'; '3'; '4'; '5'; '6'; '7'; '8'; '9'; 'A'; 'B'; 'D'; 'E'; 'F'; 'G'; 'H'; 'I'; 'J'; 'K'; 'L'; 'M'; 'N'; 'O'; 'P'; 'Q'; 'R'; 'S'; 'T'; 'U'; 'W'; 'X'; 'Y'; 'Z']  image=dspba_prim.jpg  text=fprintf('In');  style=Optimised  dataSignals=2  foldingEnabled=off  channels=ChanCount  sampleRate=SampleRate  visibilities=dspba_ChannelInVis(gcb)  version=20090408
  ChannelOut : DSPBAPrim/ChannelOut  primtype=channelout  nInputs=dspba_internal_get_channel_ports(gcb)  nOutputs=dspba_internal_get_channel_ports(gcb)  omode=Inherit via internal rule  otype=sfix(16)  scale=2^-15  rndmethod=Unbiased  factor=1  satmethod=Symmetric  shift_vec=[0 1 2 -1]  value=6  inPortNames=['v'; 'c'; '0'; '1'; '2'; '3'; '4'; '5'; '6'; '7'; '8'; '9'; 'A'; 'B'; 'D'; 'E'; 'F'; 'G'; 'H'; 'I'; 'J'; 'K'; 'L'; 'M'; 'N'; 'O'; 'P'; 'Q'; 'R'; 'S'; 'T'; 'U'; 'W'; 'X'; 'Y'; 'Z']  outPortNames=['v'; 'c'; '0'; '1'; '2'; '3'; '4'; '5'; '6'; '7'; '8'; '9'; 'A'; 'B'; 'D'; 'E'; 'F'; 'G'; 'H'; 'I'; 'J'; 'K'; 'L'; 'M'; 'N'; 'O'; 'P'; 'Q'; 'R'; 'S'; 'T'; 'U'; 'W'; 'X'; 'Y'; 'Z']  image=dspba_prim.jpg  text=fprintf('Out%s', AdvDSPBChannelOutDisplay(latency));  style=Optimised  dataSignals=6  foldingEnabled=off  channels=ChanCount  sampleRate=SampleRate  visibilities=dspba_ChannelOutVis(gcb)  latency=0  version=20090408
  CmpNE : DSPBAPrim/CmpNE  primtype=cmpne  nInputs=2  nOutputs=1  omode=boolean  otype=sfix(16)  scale=2^-15  rndmethod=Unbiased  factor=1  satmethod=Symmetric  shift_vec=[0 1 2 -1]  value=0  inPortNames=[' '; ' ';]  outPortNames=[' ']  image=dspba_prim.jpg  text=fprintf('~=');  style=Optimised  visibilities=0  version=20090407
  SampleDelay : DSPBAPrim/SampleDelay  primtype=sampdelay  nInputs=1  nOutputs=1  omode=Inherit via internal rule  otype=sfix(16)  scale=2^-15  rndmethod=Unbiased  factor=1  satmethod=Symmetric  shift_vec=[0 1 2 -1]  value=1  inPortNames=[' '; ' ';]  outPortNames=[' ']  image=dspba_prim.jpg  text=dpoly(1, eye(1,value+1), 'z')  style=Optimised  visibilities=8 + 1024  version=20090407
  SynthesisInfo : DSPBAPrim/SynthesisInfo  primtype=synthinfo  nInputs=0  nOutputs=0  omode=Inherit via internal rule  otype=sfix(16)  scale=2^-15  rndmethod=Truncate  factor=1  satmethod=Symmetric  shift_vec=[0 1 2 -1]  value=99  inPortNames=[' '; ' ';]  outPortNames=[' ']  image=dspba_prim_ctrl.jpg  text=fprintf('Style=%s', style);  style=Scheduled  visibilities=32768  constraintInUse=off  constraintRelation=>  constraintLimit=2  version=20090407
  coeff_cnt : Subsystem
  gen_coeff_offset : Subsystem
  gen_outvalid : Subsystem
  mem_cnt : Subsystem
  qv : Outport  OutDataType=sfix(16)  OutScaling=2^0
  qc : Outport  Port=2  OutDataType=sfix(16)  OutScaling=2^0
  coeff_addr : Outport  Port=3  OutDataType=sfix(16)  OutScaling=2^0
  coffset : Outport  Port=4  OutDataType=sfix(16)  OutScaling=2^0
  mem_addr : Outport  Port=5  OutDataType=sfix(16)  OutScaling=2^0
  data_out : Outport  Port=6  OutDataType=sfix(16)  OutScaling=2^0
  rate_out : Outport  Port=7  OutDataType=sfix(16)  OutScaling=2^0
  outvalid : Outport  Port=8  OutDataType=sfix(16)  OutScaling=2^0
  wires:
  v/1 -> ChannelIn/1
  c/1 -> ChannelIn/2
  ChannelOut/1 -> qv/1
  ChannelOut/2 -> qc/1
  ChannelOut/3 -> coeff_addr/1
  ChannelIn/1 -> ChannelOut/1, gen_outvalid/1(in_valid)
  rate_in/1 -> ChannelIn/3
  data_in/1 -> ChannelIn/4
  ChannelIn/2 -> ChannelOut/2
  coeff_cnt/1(coeff_cnt) -> gen_outvalid/2(coeff_cnt), ChannelOut/3  "ccnt"
  gen_coeff_offset/1(coffset) -> ChannelOut/4  "coffset"
  SampleDelay/1 -> CmpNE/1
  ChannelIn/3 -> SampleDelay/1, coeff_cnt/1(rate), CmpNE/2, mem_cnt/2(rate), ChannelOut/7
  CmpNE/1 -> coeff_cnt/2(transig), gen_coeff_offset/1(transig), mem_cnt/1(transig)  "transig"
  ChannelOut/4 -> coffset/1
  ChannelIn/4 -> ChannelOut/8
  ChannelOut/8 -> data_out/1
  ChannelOut/7 -> rate_out/1
  mem_cnt/1(mem_cnt) -> ChannelOut/6  "mcnt"
  ChannelOut/6 -> mem_addr/1
  gen_outvalid/1(out_valid) -> ChannelOut/5
  ChannelOut/5 -> outvalid/1

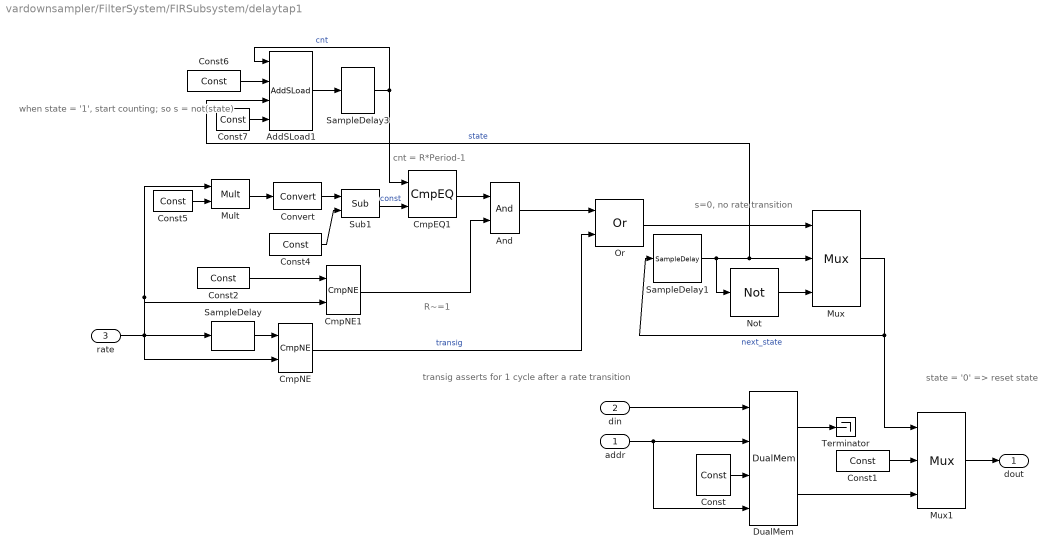
== system vardownsampler/FilterSystem/FIRSubsystem/delaytap1 ==
  note: s=0, no rate transition
  note: transig asserts for 1 cycle after a rate transition
  note: cnt = R*Period-1
  note: when state = '1', start counting;
      | so s = not(state)
  note: state = '0' => reset state
  note: R~=1
  addr : Inport
  din : Inport  Port=2
  rate : Inport  Port=3
  AddSLoad1 : DSPBAPrim/AddSLoad  primtype=addsload  nInputs=4  nOutputs=1  omode=Specify via dialog  otype=uint(resetCntWidth)  scale=1  rndmethod=Unbiased  factor=1  satmethod=Symmetric  shift_vec=[0 1 2 -1]  value=0  inPortNames=['+'; '+'; 's'; 'v']  outPortNames=[' ']  image=dspba_prim.jpg  text=fprintf('+');  style=Optimised  visibilities=8  version=20090407
  And : DSPBAPrim/And  primtype=and  nInputs=2  nOutputs=1  omode=Inherit via internal rule  otype=sfix(16)  scale=2^-15  rndmethod=Unbiased  factor=1  satmethod=Symmetric  shift_vec=[0 1 2 -1]  value=0  inPortNames=[' '; ' '; ' '; ' '; ' '; ' '; ' '; ' '; ' '; ' '; ' '; ' '; ' '; ' '; ' '; ' '; ]  outPortNames=[' ']  image=dspba_prim.jpg  text=fprintf('&');  style=Optimised  visibilities=8+2  version=20090407
  CmpEQ1 : DSPBAPrim/CmpEQ  primtype=cmpeq  nInputs=2  nOutputs=1  omode=boolean  otype=sfix(16)  scale=2^-15  rndmethod=Unbiased  factor=1  satmethod=Symmetric  shift_vec=[0 1 2 -1]  value=0  inPortNames=[' '; ' ';]  outPortNames=[' ']  image=dspba_prim.jpg  text=fprintf('==');  style=Optimised  visibilities=0  version=20090407
  CmpNE : DSPBAPrim/CmpNE  primtype=cmpne  nInputs=2  nOutputs=1  omode=boolean  otype=sfix(16)  scale=2^-15  rndmethod=Unbiased  factor=1  satmethod=Symmetric  shift_vec=[0 1 2 -1]  value=0  inPortNames=[' '; ' ';]  outPortNames=[' ']  image=dspba_prim.jpg  text=fprintf('~=');  style=Optimised  visibilities=0  version=20090407
  CmpNE1 : DSPBAPrim/CmpNE  primtype=cmpne  nInputs=2  nOutputs=1  omode=boolean  otype=sfix(16)  scale=2^-15  rndmethod=Unbiased  factor=1  satmethod=Symmetric  shift_vec=[0 1 2 -1]  value=0  inPortNames=[' '; ' ';]  outPortNames=[' ']  image=dspba_prim.jpg  text=fprintf('~=');  style=Optimised  visibilities=0  version=20090407
  Const : DSPBAPrim/Const  primtype=const  nInputs=0  nOutputs=1  omode=Inherit via internal rule  otype=sfix(16)  scale=2^-15  rndmethod=Unbiased  factor=1  satmethod=Symmetric  shift_vec=[0 1 2 -1]  value=1  inPortNames=['+'; '+';]  outPortNames=[' ']  image=dspba_prim.jpg  text=fprintf('%s', num2str(value));  style=Optimised  visibilities=8 + 1024  version=20090407
  Const1 : DSPBAPrim/Const  primtype=const  nInputs=0  nOutputs=1  omode=Specify via dialog  otype=sfix(dataWidth)  scale=2^(-dataWidth+1)  rndmethod=Unbiased  factor=1  satmethod=Symmetric  shift_vec=[0 1 2 -1]  value=0  inPortNames=['+'; '+';]  outPortNames=[' ']  image=dspba_prim.jpg  text=fprintf('%s', num2str(value));  style=Optimised  visibilities=8 + 1024  version=20090407
  Const2 : DSPBAPrim/Const  primtype=const  nInputs=0  nOutputs=1  omode=Specify via dialog  otype=uint(RateWidth)  scale=1  rndmethod=Unbiased  factor=1  satmethod=Symmetric  shift_vec=[0 1 2 -1]  value=1  inPortNames=['+'; '+';]  outPortNames=[' ']  image=dspba_prim.jpg  text=fprintf('%s', num2str(value));  style=Optimised  visibilities=8 + 1024  version=20090407
  Const4 : DSPBAPrim/Const  primtype=const  nInputs=0  nOutputs=1  omode=Specify via dialog  otype=uint(resetCntWidth)  scale=1  rndmethod=Unbiased  factor=1  satmethod=Symmetric  shift_vec=[0 1 2 -1]  value=1  inPortNames=['+'; '+';]  outPortNames=[' ']  image=dspba_prim.jpg  text=fprintf('%s', num2str(value));  style=Optimised  visibilities=8 + 1024  version=20090407
  Const5 : DSPBAPrim/Const  primtype=const  nInputs=0  nOutputs=1  omode=Specify via dialog  otype=uint(resetCntWidth)  scale=1  rndmethod=Unbiased  factor=1  satmethod=Symmetric  shift_vec=[0 1 2 -1]  value=Period  inPortNames=['+'; '+';]  outPortNames=[' ']  image=dspba_prim.jpg  text=fprintf('%s', num2str(value));  style=Optimised  visibilities=8 + 1024  version=20090407
  Const6 : DSPBAPrim/Const  primtype=const  nInputs=0  nOutputs=1  omode=Specify via dialog  otype=uint(resetCntWidth)  scale=1  rndmethod=Unbiased  factor=1  satmethod=Symmetric  shift_vec=[0 1 2 -1]  value=1  inPortNames=['+'; '+';]  outPortNames=[' ']  image=dspba_prim.jpg  text=fprintf('%s', num2str(value));  style=Optimised  visibilities=8 + 1024  version=20090407
  Const7 : DSPBAPrim/Const  primtype=const  nInputs=0  nOutputs=1  omode=Specify via dialog  otype=uint(resetCntWidth)  scale=1  rndmethod=Unbiased  factor=1  satmethod=Symmetric  shift_vec=[0 1 2 -1]  value=0  inPortNames=['+'; '+';]  outPortNames=[' ']  image=dspba_prim.jpg  text=fprintf('%s', num2str(value));  style=Optimised  visibilities=8 + 1024  version=20090407
  Convert : DSPBAPrim/Convert  primtype=convert  nInputs=1  nOutputs=1  omode=Specify via dialog  otype=uint(resetCntWidth)  scale=1  rndmethod=Truncate  factor=1  satmethod=None  shift_vec=[0 1 2 -1]  value=round([0:255]/17)  inPortNames=[' '; ' ';]  outPortNames=[' '; 'c']  image=dspba_prim.jpg  text=fprintf('convert');  style=Optimised  visibilities=8+64+256  clipdetect=off  version=20090611
  DualMem : DSPBAPrim/DualMem  primtype=dualmem  nInputs=4  nOutputs=2  omode=Inherit via internal rule  otype=sfix(16)  scale=2^-15  rndmethod=Unbiased  factor=1  satmethod=Symmetric  shift_vec=[0 1 2 -1]  value=[zeros(Nmax, 1)]  inPortNames=['d'; 'a'; 'w'; 'a']  outPortNames=['q1'; 'q2']  image=dspba_prim.jpg  text=fprintf('dmem%s',AdvDSPBDMemDisplay(UseDontCare));  style=Optimised  visibilities=8 + 1024  UseDontCare=off  version=20090407
  Mult : DSPBAPrim/Mult  primtype=mult  nInputs=2  nOutputs=1  omode=Inherit via internal rule  otype=sfix(16)  scale=2^-15  rndmethod=Unbiased  factor=1  satmethod=Symmetric  shift_vec=[0 1 2 -1]  value=0  inPortNames=[' '; ' ';]  outPortNames=[' ']  image=dspba_prim.jpg  text=fprintf('X');  style=Optimised  visibilities=8  version=20090407
  Mux : DSPBAPrim/Mux  primtype=mux  nInputs=evalAionMaskParam(gcb,'value',1)+1  nOutputs=1  omode=Inherit via internal rule  otype=sfix(16)  scale=2^-15  rndmethod=Unbiased  factor=1  satmethod=Symmetric  shift_vec=[0 1 2 -1]  value=2  inPortNames=['s'; 'd0'; 'd1'; 'd2'; 'd3'; 'd4'; 'd5'; 'd6'; 'd7'; 'd8'; 'd9';]  outPortNames=[' ']  image=dspba_prim.jpg  text=fprintf('%s', primtype);  style=Optimised  visibilities=1032  version=20090623
  Mux1 : DSPBAPrim/Mux  primtype=mux  nInputs=evalAionMaskParam(gcb,'value',1)+1  nOutputs=1  omode=Inherit via internal rule  otype=sfix(16)  scale=2^-15  rndmethod=Unbiased  factor=1  satmethod=Symmetric  shift_vec=[0 1 2 -1]  value=2  inPortNames=['s'; 'd0'; 'd1'; 'd2'; 'd3'; 'd4'; 'd5'; 'd6'; 'd7'; 'd8'; 'd9';]  outPortNames=[' ']  image=dspba_prim.jpg  text=fprintf('%s', primtype);  style=Optimised  visibilities=1032  version=20090623
  Not : DSPBAPrim/Not  primtype=not  nInputs=1  nOutputs=1  omode=Inherit via internal rule  otype=sfix(16)  scale=2^-15  rndmethod=Unbiased  factor=1  satmethod=Symmetric  shift_vec=[0 1 2 -1]  value=0  inPortNames=[' '; ' ';]  outPortNames=[' ']  image=dspba_prim.jpg  text=fprintf('~');  style=Optimised  visibilities=8  version=20090407
  Or : DSPBAPrim/Or  primtype=or  nInputs=2  nOutputs=1  omode=Inherit via internal rule  otype=sfix(16)  scale=2^-15  rndmethod=Unbiased  factor=1  satmethod=Symmetric  shift_vec=[0 1 2 -1]  value=0  inPortNames=[' '; ' '; ' '; ' '; ' '; ' '; ' '; ' '; ' '; ' '; ' '; ' '; ' '; ' '; ' '; ' '; ]  outPortNames=[' ']  image=dspba_prim.jpg  text=fprintf('|');  style=Optimised  visibilities=8+2  version=20090407
  SampleDelay : DSPBAPrim/SampleDelay  primtype=sampdelay  nInputs=1  nOutputs=1  omode=Inherit via internal rule  otype=sfix(16)  scale=2^-15  rndmethod=Unbiased  factor=1  satmethod=Symmetric  shift_vec=[0 1 2 -1]  value=1  inPortNames=[' '; ' ';]  outPortNames=[' ']  image=dspba_prim.jpg  text=dpoly(1, eye(1,value+1), 'z')  style=Optimised  visibilities=8 + 1024  version=20090407
  SampleDelay1 : DSPBAPrim/SampleDelay  primtype=sampdelay  nInputs=1  nOutputs=1  omode=boolean  otype=sfix(16)  scale=2^-15  rndmethod=Unbiased  factor=1  satmethod=Symmetric  shift_vec=[0 1 2 -1]  value=1  inPortNames=[' '; ' ';]  outPortNames=[' ']  image=dspba_prim.jpg  text=dpoly(1, eye(1,value+1), 'z')  style=Optimised  visibilities=8 + 1024  version=20090407
  SampleDelay3 : DSPBAPrim/SampleDelay  primtype=sampdelay  nInputs=1  nOutputs=1  omode=Inherit via internal rule  otype=uint(memAddrWidth)  scale=1  rndmethod=Unbiased  factor=1  satmethod=Symmetric  shift_vec=[0 1 2 -1]  value=1  inPortNames=[' '; ' ';]  outPortNames=[' ']  image=dspba_prim.jpg  text=dpoly(1, eye(1,value+1), 'z')  style=Optimised  visibilities=8 + 1024  version=20090407
  Sub1 : DSPBAPrim/Sub  primtype=sub  nInputs=2  nOutputs=1  omode=Specify via dialog  otype=uint(memAddrWidth)  scale=1  rndmethod=Unbiased  factor=1  satmethod=Symmetric  shift_vec=[0 1 2 -1]  value=0  inPortNames=['+'; '-';]  outPortNames=[' ']  image=dspba_prim.jpg  text=fprintf('-');  style=Optimised  visibilities=8  version=20090407
  Terminator : Terminator
  dout : Outport  OutDataType=fixdt(1, 16)  OutScaling=2^0
  wires:
  Mux/1 -> SampleDelay1/1, Mux1/1  "next_state"
  SampleDelay/1 -> CmpNE/1
  rate/1 -> SampleDelay/1, CmpNE/2, Mult/1, CmpNE1/2
  CmpNE/1 -> Or/2  "transig"
  Const4/1 -> Sub1/2
  Mult/1 -> Convert/1
  Sub1/1 -> CmpEQ1/2  "const"
  Const5/1 -> Mult/2
  Convert/1 -> Sub1/1
  Const6/1 -> AddSLoad1/2
  AddSLoad1/1 -> SampleDelay3/1
  SampleDelay3/1 -> AddSLoad1/1, CmpEQ1/1  "cnt"
  Const7/1 -> AddSLoad1/4
  Or/1 -> Mux/1
  SampleDelay1/1 -> AddSLoad1/3, Mux/2, Not/1  "state"
  din/1 -> DualMem/1
  addr/1 -> DualMem/2, DualMem/4
  Const/1 -> DualMem/3
  DualMem/1 -> Terminator/1
  Mux1/1 -> dout/1
  Not/1 -> Mux/3
  Const1/1 -> Mux1/2
  DualMem/2 -> Mux1/3
  Const2/1 -> CmpNE1/1
  And/1 -> Or/1
  CmpEQ1/1 -> And/1
  CmpNE1/1 -> And/2
